simulink model "dip_ekf_sim_student"  (R2017a)
settings: Solver=ode45  StartTime=0.0  StopTime=10  FixedStep=0.01  MaxStep=0.05  RelTol=1e-3  EnableMultiTasking=on
settings Model: Creator=ut  LastModifiedBy=maam
settings DataIOCC: LimitDataPoints=on  SaveFormat=Array  SignalLoggingSaveFormat=ModelDataLogs
settings OptimizationCC: ExpressionDepthLimit=2147483647  InitFltsAndDblsToZero=on  LifeSpan=inf
settings DebuggingCC: SaveWithParameterizedLinksMsg=none  UnderspecifiedInitializationDetection=Classic  MergeDetectMultiDrivingBlocksExec=none  SignalResolutionControl=TryResolveAllWithWarning  SolverPrmCheckMsg=warning  MultiTaskDSMMsg=warning  MultiTaskCondExecSysMsg=none  FcnCallInpInsideContextMsg=warning  StateNameClashWarn=warning  SFUnexpectedBacktrackingDiag=warning  SFNoUnconditionalDefaultTransitionDiag=warning  SFExecutionAtInitializationDiag=none
settings HardwareCC: ProdBitPerPointer=32  ProdBitPerSizeT=32  ProdBitPerPtrDiffT=32  ProdLargestAtomicFloat=None  ProdIntDivRoundTo=Undefined  ProdEndianess=Unspecified  ProdWordSize=32  ProdHWDeviceType=32-bit Generic
settings ModelReferenceCC: PropagateSignalLabelsOutOfModel=off
settings GRTTargetCC: TargetFcnLib=ansi_tfl_tmw.mat  TargetLangStandard=C89/C90 (ANSI)  CombineOutputUpdateFcns=off  GRTInterface=on
settings ConfigComp: CovMetricSettings=dw  CovSaveCumulativeToWorkspaceVar=on  CovSaveSingleToWorkspaceVar=on  CovExternalEMLEnable=off

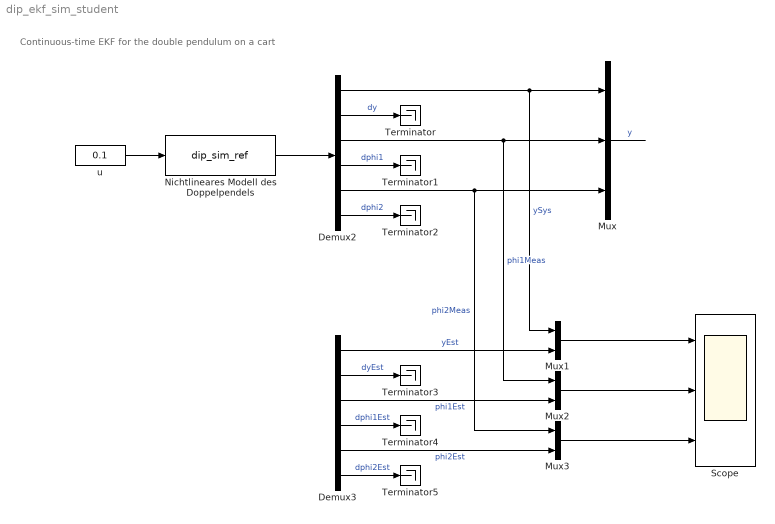
== system dip_ekf_sim_student ==
  note: Continuous-time EKF for the double pendulum on a cart
  Demux2 : Demux  Outputs=6
  Demux3 : Demux  Outputs=6
  Mux : Mux  Inputs=3
  Mux1 : Mux  Inputs=2
  Mux2 : Mux  Inputs=2
  Mux3 : Mux  Inputs=2
  Nichtlineares Modell des Doppelpendels : M-S-Function  FunctionName=dip_sim_ref  Parameters=x0
  Scope : Scope  NumInputPorts=3
  Terminator{,1..5} (6 alike) : Terminator
  u : Constant  Value=0.1
  wires:
  u/1 -> Nichtlineares Modell des Doppelpendels/1
  Nichtlineares Modell des Doppelpendels/1 -> Demux2/1
  Demux2/1 -> Mux1/1, Mux/1  "ySys"
  Demux2/3 -> Mux2/1, Mux/2  "phi1Meas"
  Demux2/5 -> Mux3/1, Mux/3  "phi2Meas"
  Demux2/2 -> Terminator/1  "dy"
  Demux2/4 -> Terminator1/1  "dphi1"
  Demux2/6 -> Terminator2/1  "dphi2"
  Demux3/5 -> Mux3/2  "phi2Est"
  Demux3/2 -> Terminator3/1  "dyEst"
  Demux3/3 -> Mux2/2  "phi1Est"
  Demux3/4 -> Terminator4/1  "dphi1Est"
  Demux3/6 -> Terminator5/1  "dphi2Est"
  Demux3/1 -> Mux1/2  "yEst"
  Mux1/1 -> Scope/1
  Mux2/1 -> Scope/2
  Mux3/1 -> Scope/3
  Mux/1 -> ?  "y"
  ? -> Demux3/1
